simulink model "extracttriang_ref"  (Simulink 4.00)
settings: Solver=FixedStepDiscrete  StartTime=0.0  StopTime=10.0  RelTol=1e-3
PostLoadFcn:
  | set_param(gcs,'SimulationCommand','Update')
libraries: dspmtrx3 x2, dspsrcs3 x1
settings Model: RequirementInfo=9  Creator=ckamachi  LastModifiedBy=ckamachi  LimitDataPoints=off  ExtModeTrigMode=oneshot  ExtModeArmWhenConnect=off  BlockReductionOpt=off

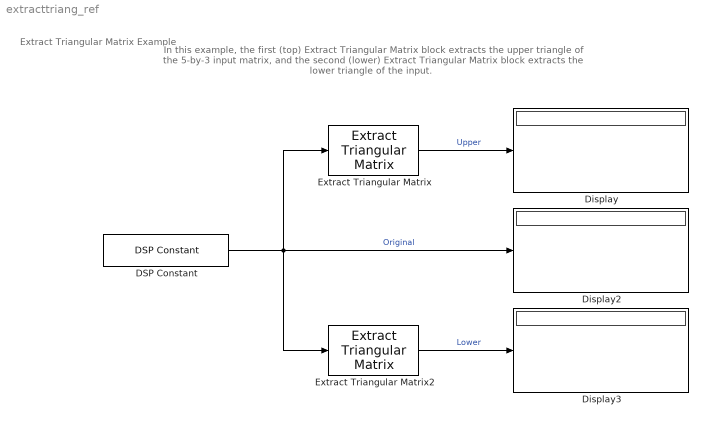
== system extracttriang_ref ==
  note: Extract Triangular Matrix Example
  note: In this example, the first (top) Extract Triangular Matrix block extracts the
      | upper triangle of the 5-by-3 input matrix, and the second (lower) Extract
      | Triangular Matrix block extracts the lower triangle of the input.
  DSP Constant : dspsrcs3/DSP Constant  Value=[1:3;4:6;7:9;10:12;13:15]  InterpretAs1D=off  SampleMode=Discrete  Ts=1  FramebasedOutput=off
  Display : Display
      settings: Format=short
  Display2 : Display
      settings: Format=short
  Display3 : Display
      settings: Format=short
  Extract Triangular Matrix : dspmtrx3/Extract Triangular Matrix  fcn=Upper
  Extract Triangular Matrix2 : dspmtrx3/Extract Triangular Matrix  fcn=Lower
  wires:
  Extract Triangular Matrix/1 -> Display/1  "Upper"
  DSP Constant/1 -> Extract Triangular Matrix2/1, Extract Triangular Matrix/1, Display2/1  "Original"
  Extract Triangular Matrix2/1 -> Display3/1  "Lower"
